simulink model "sysid"  (R2019b)
settings: Solver=ode45  StartTime=0.0  StopTime=60  RelTol=1e-3
model workspace (MAT data in the model file):
  Var = 12
values from neighbouring files (symbols this model uses):
  a = alpha(i)    [eigenplot.m]    (also in main.m; main1.m)
  h = trim(1)    [main.m]    (also in main1.m)
  q = 0    [eigenplot.m]    (also in main.m; main1.m; roots_eq.m; roots_temp.m)
libraries: simulink_extras x4, simulink x2, aerolibatmos2 x1
settings Model: NumberOfSteps=10  Creator=chenjie  LastModifiedBy=chenjie

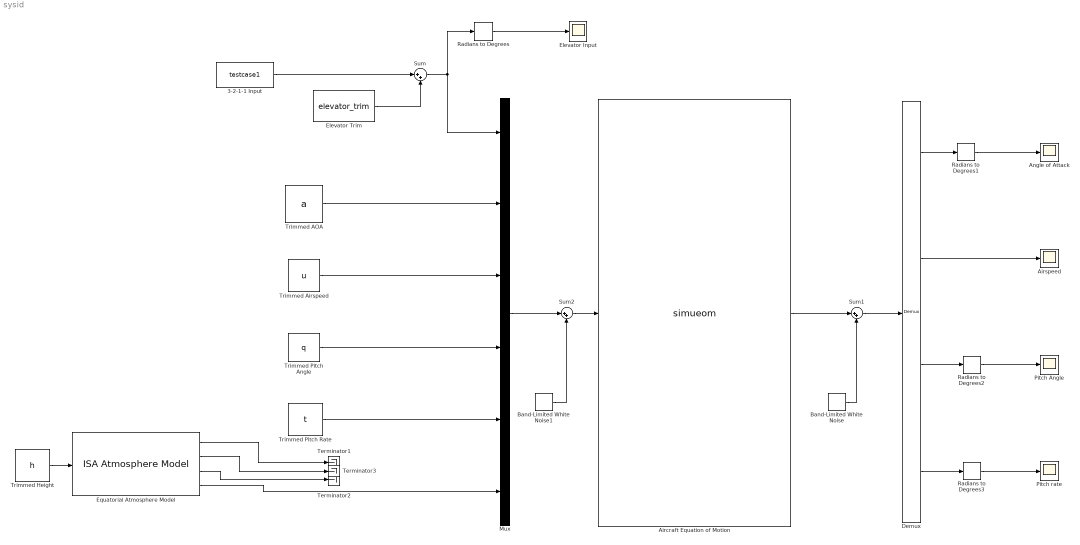
== system sysid ==
  "3-2-1-1 Input " : FromWorkspace  VariableName=testcase1  SampleTime=0
  Aircraft Equation of Motion : S-Function  FunctionName=simueom  Parameters=a,u,q,t,h  SFunctionDeploymentMode=off  EnableBusSupport=off
  Airspeed : Scope
  Angle of Attack : Scope
  Band-Limited White Noise : simulink/Sources/Band-Limited White Noise  Cov=[0.05]  Ts=0.1  seed=[23341]
  Band-Limited White Noise1 : simulink/Sources/Band-Limited White Noise  Cov=[0.05]  Ts=0.1  seed=[23341]
  Demux : Demux
  Elevator Input : Scope
  Elevator Trim : FromWorkspace  VariableName=elevator_trim  SampleTime=0
  Equatorial Atmosphere Model : aerolibatmos2/ISA Atmosphere Model  custom=on  g=9.81  gamma=1.4  R=287.0531  L=0.0065  h_trop=19000  h_strat=20000  rho0=1.165  P0=101325  T0=288.15  h0=0
      settings: SourceProductName=Aerospace Blockset
  Mux : Mux  Inputs=6
  Pitch Angle : Scope
  Pitch rate : Scope
  Radians to Degrees{,1..3} (4 alike) : simulink_extras/Transformations/Radians to Degrees
  Sum : Sum  Inputs=|++
  Sum1 : Sum  Inputs=|++
  Sum2 : Sum  Inputs=|++
  Terminator1 : Terminator
  Terminator2 : Terminator
  Terminator3 : Terminator
  "Trimmed Height " : Constant  Value=h
  "Trimmed Pitch Angle " : Constant  Value=q
  "Trimmed Pitch Rate " : Constant  Value=t
  Trimmed AOA : Constant  Value=a
  Trimmed Airspeed : Constant  Value=u
  wires:
  Elevator Trim/1 -> Sum/2
  "Trimmed Height "/1 -> Equatorial Atmosphere Model/1
  Equatorial Atmosphere Model/3 -> Terminator2/1
  Equatorial Atmosphere Model/1 -> Terminator1/1
  "3-2-1-1 Input "/1 -> Sum/1
  Radians to Degrees/1 -> Elevator Input/1
  Demux/1 -> Radians to Degrees1/1
  Sum/1 -> Mux/1, Radians to Degrees/1
  Demux/3 -> Radians to Degrees2/1
  Demux/4 -> Radians to Degrees3/1
  Trimmed Airspeed/1 -> Mux/3
  Trimmed AOA/1 -> Mux/2
  "Trimmed Pitch Rate "/1 -> Mux/5
  "Trimmed Pitch Angle "/1 -> Mux/4
  Equatorial Atmosphere Model/2 -> Terminator3/1
  Demux/2 -> Airspeed/1
  Radians to Degrees1/1 -> Angle of Attack/1
  Radians to Degrees2/1 -> Pitch Angle/1
  Radians to Degrees3/1 -> Pitch rate/1
  Equatorial Atmosphere Model/4 -> Mux/6
  Aircraft Equation of Motion/1 -> Sum1/1
  Sum1/1 -> Demux/1
  Band-Limited White Noise/1 -> Sum1/2
  Sum2/1 -> Aircraft Equation of Motion/1
  Mux/1 -> Sum2/1
  Band-Limited White Noise1/1 -> Sum2/2
